simulink model "gain_test_Ku_complex"  (Simulink 8.4)
settings: Solver=ode45  StartTime=0.0  StopTime=10.0  RelTol=1e-3
settings Model: Creator=arnaud  LastModifiedBy=arnaud
settings DataIOCC: SaveFormat=Structure

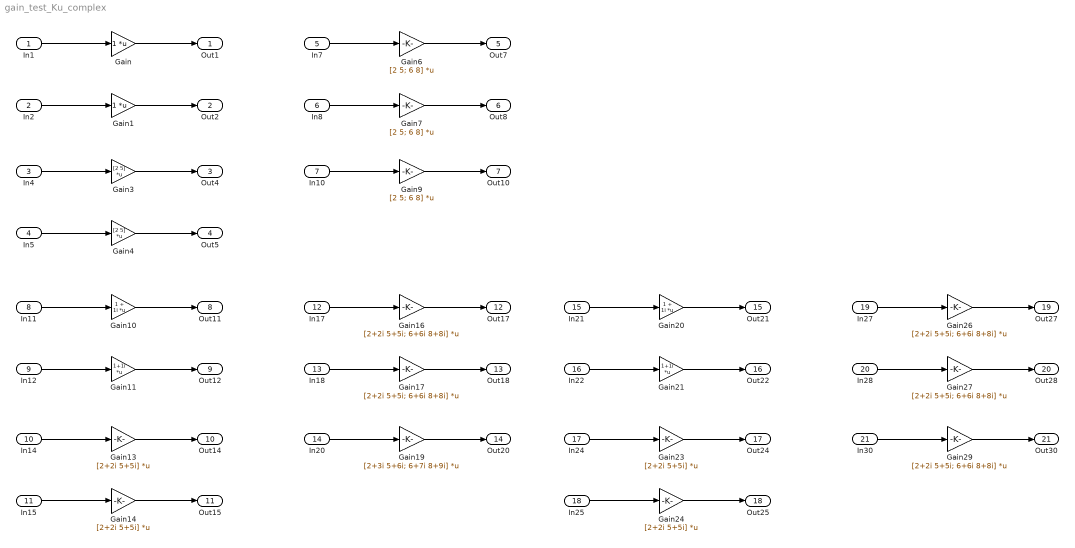
== system gain_test_Ku_complex ==
  In1 : Inport  OutDataTypeStr=double
      settings: SignalType=complex
  In2 : Inport  Port=2  OutDataTypeStr=int8
      settings: SignalType=complex
  In4 : Inport  Port=3  OutDataTypeStr=double  PortDimensions=[2 1]
      settings: SignalType=complex
  In5 : Inport  Port=4  OutDataTypeStr=int8  PortDimensions=[2 1]
      settings: SignalType=complex
  In7 : Inport  Port=5  OutDataTypeStr=double  PortDimensions=[2 1]
      settings: SignalType=complex
  In8 : Inport  Port=6  OutDataTypeStr=int8  PortDimensions=[2 1]
      settings: SignalType=complex
  In10 : Inport  Port=7  OutDataTypeStr=double  PortDimensions=[2 3]
      settings: SignalType=complex
  In11 : Inport  Port=8  OutDataTypeStr=double
      settings: SignalType=complex
  In12 : Inport  Port=9  OutDataTypeStr=int8
      settings: SignalType=complex
  In14 : Inport  Port=10  OutDataTypeStr=double  PortDimensions=[2 1]
      settings: SignalType=complex
  In15 : Inport  Port=11  OutDataTypeStr=int8  PortDimensions=[2 1]
      settings: SignalType=complex
  In17 : Inport  Port=12  OutDataTypeStr=double  PortDimensions=[2 1]
      settings: SignalType=complex
  In18 : Inport  Port=13  OutDataTypeStr=int8  PortDimensions=[2 1]
      settings: SignalType=complex
  In20 : Inport  Port=14  OutDataTypeStr=double  PortDimensions=[2 3]
      settings: SignalType=complex
  In21 : Inport  Port=15  OutDataTypeStr=double
  In22 : Inport  Port=16  OutDataTypeStr=int8
  In24 : Inport  Port=17  OutDataTypeStr=double  PortDimensions=[2 1]
  In25 : Inport  Port=18  OutDataTypeStr=int8  PortDimensions=[2 1]
  In27 : Inport  Port=19  OutDataTypeStr=double  PortDimensions=[2 1]
  In28 : Inport  Port=20  OutDataTypeStr=int8  PortDimensions=[2 1]
  In30 : Inport  Port=21  OutDataTypeStr=double  PortDimensions=[2 3]
  Gain : Gain  Multiplication=Matrix(K*u)
  Gain1 : Gain  Multiplication=Matrix(K*u)
  Gain10 : Gain  Gain=1 + 1i  Multiplication=Matrix(K*u)
  Gain11 : Gain  Gain=1+1i  Multiplication=Matrix(K*u)
  Gain{13..14,23..24} (4 alike) : Gain  Gain=[2+2i 5+5i]  Multiplication=Matrix(K*u)
  Gain{16..17,26..27,29} (5 alike) : Gain  Gain=[2+2i 5+5i; 6+6i 8+8i]  Multiplication=Matrix(K*u)
  Gain19 : Gain  Gain=[2+3i 5+6i; 6+7i 8+9i]  Multiplication=Matrix(K*u)
  Gain20 : Gain  Gain=1 + 1i  Multiplication=Matrix(K*u)
  Gain21 : Gain  Gain=1+1i  Multiplication=Matrix(K*u)
  Gain3 : Gain  Gain=[2 5]  Multiplication=Matrix(K*u)
  Gain4 : Gain  Gain=[2 5]  Multiplication=Matrix(K*u)
  Gain6 : Gain  Gain=[2 5; 6 8]  Multiplication=Matrix(K*u)
  Gain7 : Gain  Gain=[2 5; 6 8]  Multiplication=Matrix(K*u)
  Gain9 : Gain  Gain=[2 5; 6 8]  Multiplication=Matrix(K*u)
  Out1 : Outport
  Out2 : Outport  Port=2
  Out4 : Outport  Port=3
  Out5 : Outport  Port=4
  Out7 : Outport  Port=5
  Out8 : Outport  Port=6
  Out10 : Outport  Port=7
  Out11 : Outport  Port=8
  Out12 : Outport  Port=9
  Out14 : Outport  Port=10
  Out15 : Outport  Port=11
  Out17 : Outport  Port=12
  Out18 : Outport  Port=13
  Out20 : Outport  Port=14
  Out21 : Outport  Port=15
  Out22 : Outport  Port=16
  Out24 : Outport  Port=17
  Out25 : Outport  Port=18
  Out27 : Outport  Port=19
  Out28 : Outport  Port=20
  Out30 : Outport  Port=21
  wires:
  In1/1 -> Gain/1
  Gain/1 -> Out1/1
  In2/1 -> Gain1/1
  Gain1/1 -> Out2/1
  In4/1 -> Gain3/1
  Gain3/1 -> Out4/1
  In5/1 -> Gain4/1
  Gain4/1 -> Out5/1
  In7/1 -> Gain6/1
  Gain6/1 -> Out7/1
  In8/1 -> Gain7/1
  Gain7/1 -> Out8/1
  In10/1 -> Gain9/1
  Gain9/1 -> Out10/1
  In11/1 -> Gain10/1
  Gain10/1 -> Out11/1
  In12/1 -> Gain11/1
  Gain11/1 -> Out12/1
  In14/1 -> Gain13/1
  Gain13/1 -> Out14/1
  In15/1 -> Gain14/1
  Gain14/1 -> Out15/1
  In17/1 -> Gain16/1
  Gain16/1 -> Out17/1
  In18/1 -> Gain17/1
  Gain17/1 -> Out18/1
  In20/1 -> Gain19/1
  Gain19/1 -> Out20/1
  In21/1 -> Gain20/1
  Gain20/1 -> Out21/1
  In22/1 -> Gain21/1
  Gain21/1 -> Out22/1
  In24/1 -> Gain23/1
  Gain23/1 -> Out24/1
  In25/1 -> Gain24/1
  Gain24/1 -> Out25/1
  In27/1 -> Gain26/1
  Gain26/1 -> Out27/1
  In28/1 -> Gain27/1
  Gain27/1 -> Out28/1
  In30/1 -> Gain29/1
  Gain29/1 -> Out30/1
